simulink model "robotwithqdes"  (R2021b)
settings: Solver=FixedStepAuto  StartTime=0.0  StopTime=5  FixedStep=1e-3  RelTol=1e-3
values from neighbouring files (symbols this model uses):
  fext = zeros(6,8)    [simIRB120_trajtracking.m]
  kd = [  20;   10;   10;  0.5;   0.5; 0.05]    [simIRB120_trajtracking.m]
  ki = [  65;   20;  300;   .5;   0.5;   .1]    [simIRB120_trajtracking.m]
  kp = [  20;  3000000;  450; 3.55;     5;  .75]    [simIRB120_trajtracking.m]
  q_table = qdes    [simIRB120_trajtracking.m]
  qdotinit = zeros(6,1)    [simIRB120_trajtracking.m]
  qinit = zeros(6,1)    [simIRB120_trajtracking.m]
  t_table = (0:.1:Tf)    [simIRB120_trajtracking.m]
  x = pinv(A)*tau_g    [gravident.m]    (also in simIRB120_trajtracking.m = [-17.0122   -3.0550   -5.6141    0.0007   -0.0846   -3.0546 )
libraries: robotmaniplib x2, slpidlib x1
settings Model: Creator=wen  LastModifiedBy=wen
settings SolverCC: AlgebraicLoopSolver=TrustRegion
settings DebuggingCC: SFMachineParentedDataDiag=warning

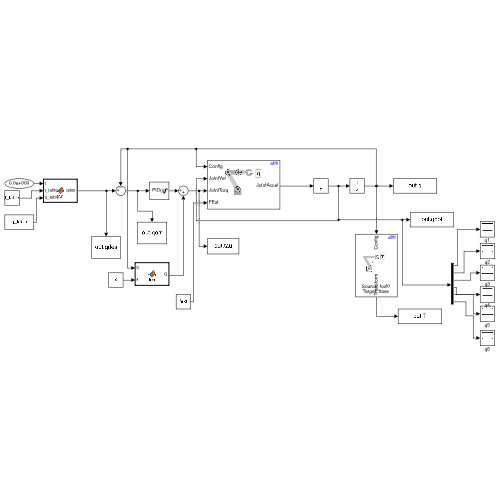
[thumbnail: Simulink's stored preview of the top-level diagram]
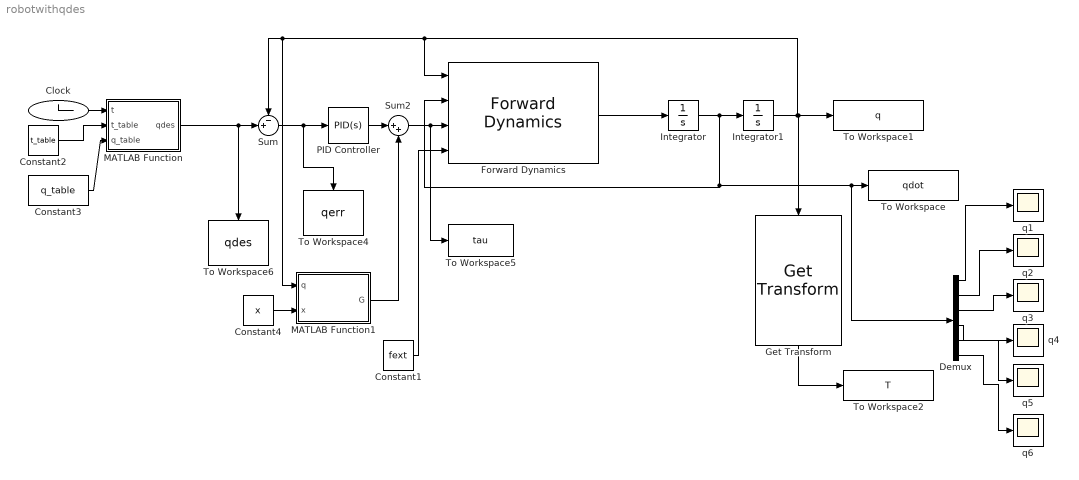
== system robotwithqdes ==
  Clock : Clock
  Constant1 : Constant  Value=fext
  Constant2 : Constant  Value=t_table
  Constant3 : Constant  Value=q_table
  Constant4 : Constant  Value=x
  Demux : Demux  Outputs=6
  Forward Dynamics : robotmaniplib/Forward Dynamics  RigidBodyTree=abb  SimulateUsing=Interpreted execution
  Get Transform : robotmaniplib/Get Transform  RigidBodyTree=abb  SourceBody=tool0  TargetBody=base  SimulateUsing=Interpreted execution
  Integrator : Integrator  InitialCondition=qdotinit
  Integrator1 : Integrator  InitialCondition=qinit
  MATLAB Function : MATLAB Function  TreatAsAtomicUnit=on
  MATLAB Function1 : MATLAB Function  TreatAsAtomicUnit=on
  PID Controller : slpidlib/PID Controller  Controller=PID  Form=Parallel  TimeDomain=Continuous-time  UseExternalTs=off  SampleTime=-1  IntegratorMethod=Forward Euler  FilterMethod=Forward Euler  ControllerParametersSource=internal  P=kp  I=ki  D=kd  UseFilter=on  N=100  TunerSelectOption=Transfer Function Based (PID Tuner App)  InitialConditionSource=internal  InitialConditionForIntegrator=0  InitialConditionForFilter=0  DifferentiatorICPrevScaledInput=0  ExternalReset=none  TrackingMode=off  Kt=1  LimitOutput=on  SatLimitsSource=internal  UpperSaturationLimit=[20;20;20;5;5;5]*.5  LowerSaturationLimit=-[20;20;20;5;5;5]*.5  LinearizeAsGain=on  AntiWindupMode=none  Kb=1  POutMin=[]  POutMax=[]  IOutMin=[]  IOutMax=[]  DOutMin=[]  DOutMax=[]  NOutMin=[]  NOutMax=[]  SumOutMin=[]  SumOutMax=[]  SaturationOutMin=[]  SaturationOutMax=[]  PParamMin=[]  PParamMax=[]  IParamMin=[]  IParamMax=[]  DParamMin=[]  DParamMax=[]  NParamMin=[]  NParamMax=[]  KbParamMin=[]  KbParamMax=[]  KtParamMin=[]  KtParamMax=[]  KbOutMin=[]  KbOutMax=[]  KtOutMin=[]  KtOutMax=[]  IntegratorOutMin=[]  IntegratorOutMax=[]  FilterOutMin=[]  FilterOutMax=[]  SumI1OutMin=[]  SumI1OutMax=[]  SumI2OutMin=[]  SumI2OutMax=[]  SumI3OutMin=[]  SumI3OutMax=[]  SumI4OutMin=[]  SumI4OutMax=[]  SumDOutMin=[]  SumDOutMax=[]  DifferentiatorOutMin=[]  DifferentiatorOutMax=[]  FilterDiffOutCoefMin=[]  FilterDiffOutCoefMax=[]  ReciprocalOutMin=[]  ReciprocalOutMax=[]  SumDenOutMin=[]  SumDenOutMax=[]  SumNumOutMin=[]  SumNumOutMax=[]  DivideOutMin=[]  DivideOutMax=[]  UdiffTsProdOutMin=[]  UdiffTsProdOutMax=[]  NTsProdOutMin=[]  NTsProdOutMax=[]  UintegralTsProdOutMin=[]  UintegralTsProdOutMax=[]  UngainTsProdOutMin=[]  UngainTsProdOutMax=[]  IntegratorContinuousStateAttributes=''  IntegratorStateMustResolveToSignalObject=off  IntegratorRTWStateStorageClass=Auto  FilterContinuousStateAttributes=''  FilterStateMustResolveToSignalObject=off  FilterRTWStateStorageClass=Auto  ParallelPVariant=InternalParameters  IdealPVariant=Disabled  IVariant=InternalParameters  DVariant=InternalParameters  IntegratorVariant=Continuous  SatVariant=Enabled  AWVariant=Passthrough  PCopyVariant=Disabled  TRVariant=Disabled  FdbkBlocksVariant=Forward  IdealPFdbkVariant=Disabled  SatFdbkVariant=Disabled  DerivativeFilterVariant=ContFilter  NVariant=InternalParameters  NCopyVariant=Disabled  FilterICVariant=InternalICsFilter  IntegratorICVariant=InternalICs  ExternalResetVariant=Disabled  TRSumVariant=Passthrough  SumFdbkVariant=Disabled  SumVariant=Sum_PID  TsampFilterVariant=InternalTs  TsampNgainVariant=Passthrough  TsampIntegralVariant=Passthrough  ExternalSaturationOutDataTypeStr=Inherit: Same as second input
  Sum : Sum  Inputs=-+|
  Sum2 : Sum  Inputs=|++
  To Workspace : ToWorkspace  VariableName=qdot  SampleTime=-1
  To Workspace1 : ToWorkspace  VariableName=q  SampleTime=-1
  To Workspace2 : ToWorkspace  VariableName=T  SampleTime=-1
  To Workspace4 : ToWorkspace  VariableName=qerr  SampleTime=-1
  To Workspace5 : ToWorkspace  VariableName=tau  SampleTime=-1
  To Workspace6 : ToWorkspace  VariableName=qdes  SampleTime=-1
  q{1..6} (6 alike) : Scope
  wires:
  Forward Dynamics/1 -> Integrator/1
  Integrator/1 -> Forward Dynamics/2, Demux/1, To Workspace/1, Integrator1/1
  Integrator1/1 -> To Workspace1/1, Get Transform/1, MATLAB Function1/1(q), Sum/1, Forward Dynamics/1
  Sum2/1 -> To Workspace5/1, Forward Dynamics/3
  Sum/1 -> To Workspace4/1, PID Controller/1
  PID Controller/1 -> Sum2/1
  Get Transform/1 -> To Workspace2/1
  MATLAB Function/1(qdes) -> To Workspace6/1, Sum/2
  Constant4/1 -> MATLAB Function1/2(x)
  MATLAB Function1/1(G) -> Sum2/2
  Demux/6 -> q6/1
  Demux/4 -> q4/1
  Demux/2 -> q2/1
  Demux/1 -> q1/1
  Demux/5 -> q5/1
  Demux/3 -> q3/1
  Constant1/1 -> Forward Dynamics/4
  Clock/1 -> MATLAB Function/1(t)
  Constant2/1 -> MATLAB Function/2(t_table)
  Constant3/1 -> MATLAB Function/3(q_table)

== matlab function robotwithqdes/MATLAB Function ==
  data: t input; qdes output; t_table input; q_table input
function qdes = fcn(t,t_table,q_table)

qdes=interp1(t_table,q_table,t)';

end

== matlab function robotwithqdes/MATLAB Function1 ==
  data: q input; G output; x input
function G = fcn(q,x)

s2=sin(q(2));
s23=sin(q(2)+q(3));
c23=cos(q(2)+q(3));
s4=sin(q(4));
c4=cos(q(4));
s5=sin(q(5));
c5=cos(q(5));

nx=12;
Aq=[zeros(1,nx);
    s2 s23 c23 s23*c4*s5 c23*c5 zeros(1,nx-5);...
    zeros(1,5) s23 c23 s23*c4*s5 c23*c5 zeros(1,nx-9);...
    zeros(1,9) c23*s4*s5 zeros(1,nx-10);...
    zeros(1,10) s23*s5 c23*c4*c5;...
    zeros(1,nx)];

G = Aq*x;

end
